simulink model "finalproj"  (R2021a)
settings: Solver=VariableStepAuto  StartTime=0.0  StopTime=inf  RelTol=1e-3
libraries: vrlib x1
settings Model: Creator=Al ien  LastModifiedBy=Al ien

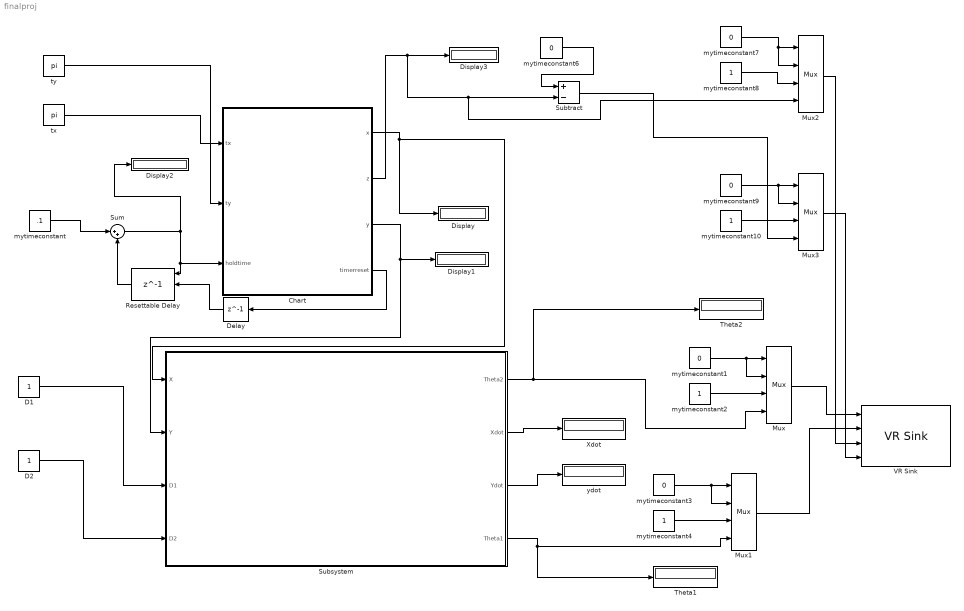
== system finalproj ==
  Chart : Stateflow chart  TreatAsAtomicUnit=on
  D1 : Constant
  D2 : Constant
  Delay : Delay  DelayLength=1  InitialCondition=0
  Display{,1..3} (4 alike) : Display
  Mux{,1..3} (4 alike) : Mux
  Resettable Delay : Delay  DelayLength=1  InitialConditionSource=Input port  ExternalReset=Rising
      settings: InputPortMap=u0,r5,p4
  Subsystem : Subsystem
  Subtract : Sum  Inputs=+-
  Sum : Sum  Inputs=|++
  Theta1 : Display
  Theta2 : Display
  VR Sink : vrlib/VR Sink  InstantiateOnLoad=on  SampleTime=0.1  ViewEnable=on  RemoteChange=off  RemoteView=off  FieldsWritten=shoulderjoint.rotation.4.1.1.double#elbowjnt.rotation.4.1.1.double#wrist.rotation.4.1.1.double#wrist2.rotation.4.1.1.double  WorldFileName=C:\Users\Al ien\Desktop\finalProj.wrl  AutoView=off  VideoDimensions=[]  AllowVariableSize=off  FigureProperties="{'Position', 'Name', 'Viewpoint', 'CameraBound', 'CameraDirection', 'CameraPosition', 'CameraUpVector', 'ZoomFactor', 'Antialiasing', 'Headlight', 'Lighting', 'NavPanel', 'Sound', 'StatusBar', 'Stereo3D', 'Stereo3DCameraOffset', 'Stereo3DHIT', 'ToolBar', 'Textures', 'Transparency', 'Triad', 'Wireframe', 'NavZones', 'NavMode', 'NavSpeed', 'CaptureFileFormat', 'CaptureFileName', 'Record2DCompressMethod', 'Record2DCompressQuality', 'Record2D', 'Record2DFileName', 'Record2DFPS'; [6.4800000000000000e+02   1.7300000000000000e+02   5.7600000000000000e+02   3.5000000000000000e+02], '', '', 'on', [2.9107725308059513e-02   0.0000000000000000e+00  -9.9957628039454316e-01], [-8.2173768748490783e-01   1.5370922088623047e+00   3.8218951925066662e+01], [0.0000000000000000e+00   1.0000000000000000e+00   0.0000000000000000e+00], [1.0000000000000000e+00], 'on', 'on', 'on', 'halfbar', 'on', 'on', 'off', [1.0000000149011612e-01], [0.0000000000000000e+00], 'on', 'on', 'on', 'none', 'off', 'off', 'fly', 'normal', 'tif', '%f_anim_%n.tif', 'auto', [7.5000000000000000e+01], 'off', '%f_anim_%n.avi', 'auto'}"
  Xdot : Display
  mytimeconstant : Constant  Value=.1
  mytimeconstant{1,3,6..7,9} (5 alike) : Constant  Value=0
  mytimeconstant{2,4,8,10} (4 alike) : Constant
  tx : Constant  Value=pi
  ty : Constant  Value=pi
  ydot : Display
  wires:
  Sum/1 -> Chart/3(holdtime), Resettable Delay/1, Display2/1
  Delay/1 -> Resettable Delay/2
  Chart/1(x) -> Display/1, Subsystem/1(X)
  Resettable Delay/1 -> Sum/2
  Chart/4(timerreset) -> Delay/1
  Chart/3(y) -> Subsystem/2(Y), Display1/1
  mytimeconstant/1 -> Sum/1
  Subsystem/2(Xdot) -> Xdot/1
  Subsystem/4(Theta1) -> Theta1/1, Mux1/4
  Subsystem/3(Ydot) -> ydot/1
  D2/1 -> Subsystem/4(D2)
  D1/1 -> Subsystem/3(D1)
  mytimeconstant2/1 -> Mux/3
  mytimeconstant1/1 -> Mux/2, Mux/1
  mytimeconstant4/1 -> Mux1/3
  mytimeconstant3/1 -> Mux1/2, Mux1/1
  Mux/1 -> VR Sink/1
  Mux1/1 -> VR Sink/2
  Subsystem/1(Theta2) -> Mux/4, Theta2/1
  ty/1 -> Chart/2(ty)
  tx/1 -> Chart/1(tx)
  mytimeconstant8/1 -> Mux2/3
  mytimeconstant7/1 -> Mux2/2, Mux2/1
  Mux2/1 -> VR Sink/3
  mytimeconstant10/1 -> Mux3/3
  mytimeconstant9/1 -> Mux3/2, Mux3/1
  Mux3/1 -> VR Sink/4
  mytimeconstant6/1 -> Subtract/1
  Subtract/1 -> Mux3/4
  Chart/2(z) -> Mux2/4, Subtract/2, Display3/1

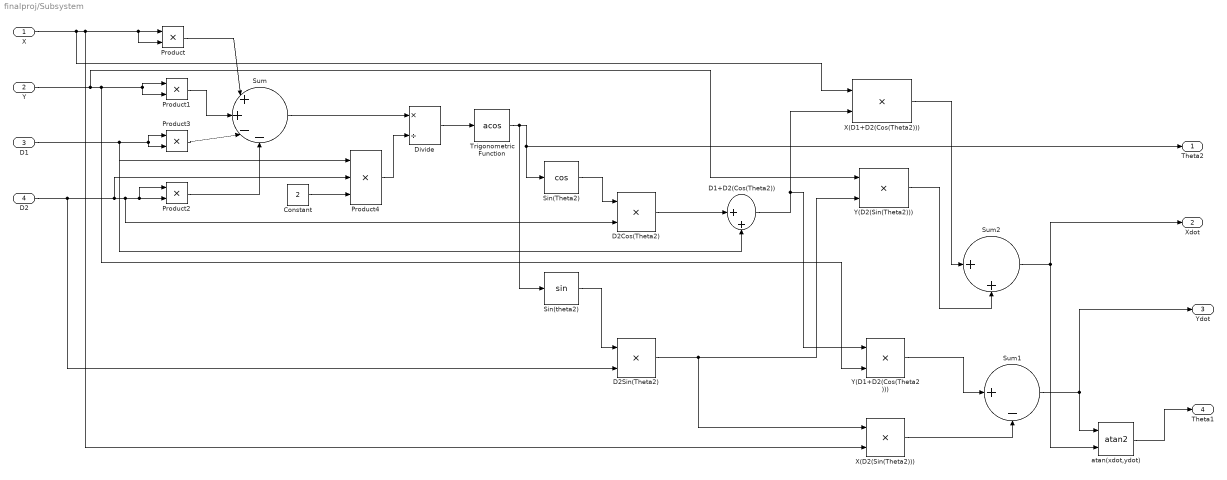
== system finalproj/Subsystem ==
  X : Inport
  Y : Inport  Port=2
  D1 : Inport  Port=3
  D2 : Inport  Port=4
  Constant : Constant  Value=2
  D1+D2(Cos(Theta2)) : Sum  Inputs=|++
  D2Cos(Theta2) : Product
  D2Sin(Theta2) : Product
  Divide : Product  Inputs=*/
  Product{,1..3} (4 alike) : Product
  Product4 : Product  Inputs=3
  Sin(Theta2) : Trigonometry  Operator=cos
  Sin(theta2) : Trigonometry
  Sum : Sum  Inputs=|++--
  Sum1 : Sum  Inputs=|+-
  Sum2 : Sum  Inputs=|++
  Trigonometric Function : Trigonometry  Operator=acos
  X(D1+D2(Cos(Theta2))) : Product
  X(D2(Sin(Theta2))) : Product
  Y(D1+D2(Cos(Theta2))) : Product
  Y(D2(Sin(Theta2))) : Product
  atan(xdot,ydot) : Trigonometry  Operator=atan2
  Theta2 : Outport
  Xdot : Outport  Port=2
  Ydot : Outport  Port=3
  Theta1 : Outport  Port=4
  wires:
  D2Sin(Theta2)/1 -> X(D2(Sin(Theta2)))/1, Y(D2(Sin(Theta2)))/2
  Product1/1 -> Sum/2
  Sum/1 -> Divide/1
  Divide/1 -> Trigonometric Function/1
  Product/1 -> Sum/1
  Sin(theta2)/1 -> D2Sin(Theta2)/1
  D1+D2(Cos(Theta2))/1 -> Y(D1+D2(Cos(Theta2)))/1, X(D1+D2(Cos(Theta2)))/2
  Product4/1 -> Divide/2
  Product3/1 -> Sum/3
  Y(D2(Sin(Theta2)))/1 -> Sum2/2
  Y(D1+D2(Cos(Theta2)))/1 -> Sum1/1
  D1/1 -> D1+D2(Cos(Theta2))/2, Product3/2, Product3/1, Product4/1
  D2/1 -> D2Sin(Theta2)/2, Product4/2, D2Cos(Theta2)/2, Product2/1, Product2/2
  X/1 -> X(D1+D2(Cos(Theta2)))/1, X(D2(Sin(Theta2)))/2, Product/2, Product/1
  Sum1/1 -> Ydot/1, atan(xdot,ydot)/1
  Sin(Theta2)/1 -> D2Cos(Theta2)/1
  Sum2/1 -> Xdot/1, atan(xdot,ydot)/2
  X(D2(Sin(Theta2)))/1 -> Sum1/2
  Trigonometric Function/1 -> Sin(theta2)/1, Theta2/1, Sin(Theta2)/1
  Y/1 -> Y(D2(Sin(Theta2)))/1, Y(D1+D2(Cos(Theta2)))/2, Product1/1, Product1/2
  X(D1+D2(Cos(Theta2)))/1 -> Sum2/1
  D2Cos(Theta2)/1 -> D1+D2(Cos(Theta2))/1
  Product2/1 -> Sum/4
  Constant/1 -> Product4/3
  atan(xdot,ydot)/1 -> Theta1/1

== stateflow chart finalproj/Chart ==
  state startstate
    x=0; y=0; z=0; timerreset=0;
  state resettimerstate
    x=0; y=0; z=0; timerreset=1;
  state centerstate
    x=0; y=0; z=0; timerreset=0;
  state outerstatetransition
    x=x+0.01; y=y+0.01; z=0; timerreset=0;
  state centerstateback
    x=0; y=0; z=0; timerreset=0;
  state outerstate
    x=tx; y=ty; z=0; timerreset=0;
  state centerstatetransition
    x=x-0.01; y=y-0.01; z=0; timerreset=0;
  state grab2
    z=0; x=tx; y=ty; timerreset=0;
  state grabtransition
    z=z+0.1; x=tx; y=ty; timerreset=0;
  state grabtransition1
    z=z-0.1; x=tx; y=ty; timerreset=0;
  state hold
    z=.3; x=tx; y=ty; timerreset=0;
  (default) -> startstate
  startstate -> centerstate
  resettimerstate -> centerstate
  centerstateback -> resettimerstate : [holdtime>250]
  centerstate -> outerstatetransition : [holdtime>25]
  outerstatetransition -> outerstate : [x>=tx && y>= ty]
  centerstatetransition -> centerstateback : [x<=pi/2 && y<=pi/2]
  outerstate -> grabtransition : [holdtime>100]
  grab2 -> centerstatetransition
  grabtransition1 -> grab2 : [z<=0]
  grabtransition -> hold : [z<=10]
  hold -> grabtransition1 : [holdtime>175]
  data: tx input; ty input; x output; z output; y output; holdtime input; timerreset output
